simulink model "raspberrypi_external_mode"  (R2018b)
settings: Solver=ode3  StartTime=0.0  StopTime=inf  RelTol=1e-3
undefined symbols (not defined in the file or in its folder): Green, led0
libraries: embdlinuxlib x1, simulink x1, realtime_examples_misc x1
settings Model: FPTRunName=Active  SimulationMode=external  ExtModeTrigDuration=2  Creator=The MathWorks, Inc.  LastModifiedBy=The MathWorks, Inc.
settings SolverCC: PositivePriorityOrder=on
settings DataIOCC: LimitDataPoints=on  SaveFormat=Array
settings OptimizationCC: ExpressionDepthLimit=2147483647  LifeSpan=Inf  MaxStackSize=64
settings DebuggingCC: UnderspecifiedInitializationDetection=Classic  MergeDetectMultiDrivingBlocksExec=none  FcnCallInpInsideContextMsg=warning  AllowSymbolicDim=off  StateNameClashWarn=warning  SFUnexpectedBacktrackingDiag=warning  SFNoUnconditionalDefaultTransitionDiag=warning  SFExecutionAtInitializationDiag=none
settings HardwareCC: ProdBitPerPointer=32  ProdBitPerSizeT=32  ProdBitPerPtrDiffT=32  ProdLargestAtomicInteger=Long  ProdLargestAtomicFloat=Double  ProdWordSize=32  ProdHWDeviceType=ARM Compatible->ARM Cortex  UseEmbeddedCoderFeatures=off  UseSimulinkCoderFeatures=off
settings ModelReferenceCC: PropagateSignalLabelsOutOfModel=off
settings SFSimCC: SimUseLocalCustomCode=off
settings RTWCC: SystemTargetFile=ert.tlc  HardwareBoard=Raspberry Pi  TemplateMakefile=ert_default_tmf  RTWVerbose=off  RTWUseLocalCustomCode=off  Toolchain=GNU GCC Raspberry Pi
settings CodeAppCC: StateflowObjectComments=on
settings ERTTargetCC: MultiwordLength=2048  ERTCustomFileBanners=off  SupportContinuousTime=on  SupportNonInlinedSFcns=on  RemoveResetFunc=off  ModelStepFunctionPrototypeControlCompliant=off  ConvertIfToSwitch=off  SuppressUnreachableDefaultCases=off
settings ConfigComp: CovMetricSettings=dw  CovHtmlReporting=on  CovSaveCumulativeToWorkspaceVar=on  CovSaveSingleToWorkspaceVar=on  CovExternalEMLEnable=off  CovSFcnEnable=off

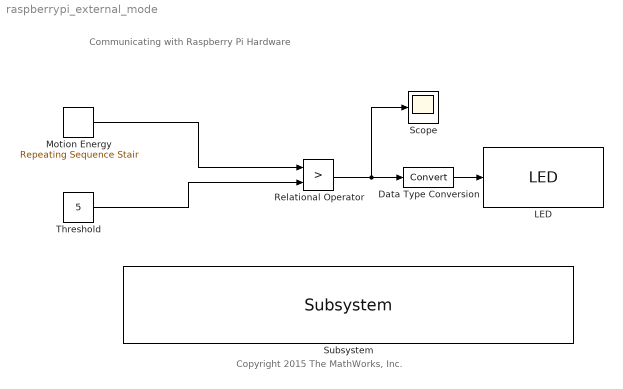
== system raspberrypi_external_mode ==
  note: Communicating with Raspberry Pi Hardware
  note: Copyright 2015 The MathWorks, Inc.
  Data Type Conversion : DataTypeConversion
  LED : embdlinuxlib/LED  board=Pi 2 Model B  led=led0 (Green)  blockPlatform=Raspberry Pi
      settings: SourceProductName=Simulink Support Package for Raspberry Pi Hardware  SourceProductBaseCode=RASPPI
  Motion Energy : simulink/Sources/Repeating Sequence Stair  OutValues=|  tsamp=0.1  OutMin=[]  OutMax=[]  OutDataTypeStr=uint8  OutputDataTypeScalingMode=uint8  OutDataType=fixdt(0,8)  ConRadixGroup=Best Precision: Vector-wise  OutScaling=2^-12
      | [ 3
      |     2
      |     2
      |     1
      |     1
      |     1
      |     1
      |     1
      |     1
      |     1
      |     1
      |     1
      |     1
      |     2
      |     3
      |     3
      |     4
      |     4
      |     5
      |     5
      |     5
      |     6
      |     5
      |     6
      |     6
      |     6
      |     7
      |     8
      |     8
      |     8
      |     9
      |     9
      |     9
      |     9
      |     9
      |    10
      |    12
      |    12
      |    11
      |    10
      |    10
      |     9
      |     8
      |     7
      |     5
      |     6
      |     5
      |     4
      |     4
      |     5
      |     5
      |     4
      |     4
      |     4
      |     3
      |     3
      |     2
      |     2
      |     2
      |     2
      |     2
      |     2
      |     2
      |     2
      |     2
      |     2
      |     1
      |     1
      |     2
      |     2
      |     2
      |     1
      |     2
      |     2
      |     2
      |     2
      |     2
      |     2
      |     2
      |     2
      |     2
      |     2
      |     2
      |     3
      |     2
      |     2
      |     3
      |     3
      |     3
      |     4
      |     4
      |     4
      |     4
      |     4
      |     4
      |     4
      |     4
      |     4
      |     4
      |     7
      |     4
      |     42
      |    39
      |     46
      |     6
      |     6
      |     7
      |     6
      |     6
      |     5
      |     5
      |     4
      |     4
      |     5
      |     5
      |     6
      |    53
      |     47
      |     50
      |     5
      |     5
      |     5
      |     6
      |     7
      |     8
      |     7
      |     7
      |     6
      |     6
      |     7
      |     8
      |     9
      |    19
      |     8
      |     8
      |     6
      |     6
      |     5
      |     5
      |     5
      |     4
      |     4
      |     4
      |     4
      |     4
      |     5
      |    17
      |     5
      |     4
      |     4]'
  Relational Operator : RelationalOperator  Operator=>  OutDataTypeStr=fixdt(1,16)  RndMeth=Nearest
  Scope : Scope
  Subsystem : realtime_examples_misc/Subsystem  SystemSampleTime=-1
  "Threshold " : Constant  Value=5  OutDataTypeStr=uint8  SampleTime=0.1
  wires:
  Motion Energy/1 -> Relational Operator/1
  Relational Operator/1 -> Data Type Conversion/1, Scope/1
  "Threshold "/1 -> Relational Operator/2
  Data Type Conversion/1 -> LED/1
